simulink model "SIM_EXO_DAL_MN"  (R2021b)
settings: Solver=VariableStepAuto  StartTime=0.0  StopTime=60  FixedStep=0.0001  RelTol=1e-4
undefined symbols (not defined in the file): b, dq, q, X, Y, Z
libraries: sm_lib x47, nesl_utility x7
(part 24 of 24)

== matlab function SIM_EXO_DAL_MN/PD+g(DIN)/MATLAB Function ==
  data: H input; ts input; b input; Kp output; Kd output
function [Kp, Kd] = ganancias(H,ts,b)
Kp = zeros(6,1);
Kd = zeros(6,1);

wn = 6/ts;

for i = 1:6
    Kp(i) = H(i,i)*(wn^2);
    Kd(i) = H(i,i)*(2*(wn^2))-b(i);
end
